simulink library "THAMO_6x2"  (R2018a)
settings: Solver=VariableStepAuto  StartTime=0.0  StopTime=10.0  RelTol=1e-3
undefined symbols (not defined in the file): BM, DiameterLastPiece, DPConstant, DPLinear, DPQuadratic, GeodeticHeight, ID, magnitude, MassFlow, Pressure, Temperature, Water
libraries: carnot x11, simulink x10, $bdroot x3
(part 2 of 3)

== system THAMO_6x2/TVL-Regler mit Hysterese ==
  note: Hystereseregler
      |
      | Erzeuger wird zwischen 0 und 1 mit Hysterese stufig geschalten
  note: Vorlauftemperaturregler
      |
      | Sollvorlauftemperatur wird aus Außentemperatur berechnet, lineares Verhalten zwischen TVLmax bei -16°C und TVLmin bei 20°C (bzw. auch über beide Grenzen hinaus)
  note: Regler Mindestmassenstrom
      |
      | Stellsignal wird nur weitergegeben wenn Massenstrom über Mindestmassenstrom liegt
  note: Reglereinheit Mindestlaufzeit
      |
      | Funktion
      | Maximalwert von Reglerausgang PID und Mindestlaufzeitregler wird gewählt
      | Wert wird geprüft und einem Betriebszustand zugeordnet (1-AN / 0-AUS)
      | IST-Betriebszustand wird integriert - Integrator wird zurückgesetzt, wenn Mindestlaufzeit erreicht
      | Abfrage Wert Integrator, wenn Integrator = 0, wird Stellsignal PID weitergegeben, das =0 sein kann, wenn Mindestlaufzeit nicht erreicht wird Minimalstellsignal ausgegeben
      |
      | Nachteil
      | - Integrator stellt sich immer nach tmin zurück, was dazu führt, dass der Regler immer mindestens tmin als Nachlaufzeit ausgibt
  t_a : Inport
  THB_VL : Inport  Port=2
  Bus Selector : BusSelector  OutputSignals=MassFlow,Temperature
  Compare To Constant : simulink/Logic and Bit Operations/Compare To Constant  relop=>=  const=mmin  OutDataTypeStr=boolean
  Constant : Constant  Value=TVLmax
  Constant1 : Constant  Value=TVLmin
  Constant2 : Constant
  Constant3 : Constant  Value=0
  Constant4 : Constant
  Constant5 : Constant  Value=0
  Constant6 : Constant  Value=T_HG
  Constant7 : Constant
  Integrator : Integrator  ExternalReset=level hold
  Memory : Memory  InitialCondition=1
  MinMax : MinMax  Function=max  Inputs=2
  MinMax1 : MinMax  Function=max  Inputs=2
  Product : Product
  Relay : Relay  OnSwitchValue=hyst_min/2  OffSwitchValue=-hyst_min/2
  Sum : Sum  Inputs=-+|
  Switch1 : Switch  Criteria=u2 > Threshold
  Switch2 : Switch  Threshold=tmin*60
  Switch3 : Switch  Threshold=tmin*60
  Switch4 : Switch  Criteria=u2 > Threshold
  TVL-Regler nach t_a : MATLAB Function  TreatAsAtomicUnit=on
  St : Outport
  wires:
  Memory/1 -> Integrator/2
  Sum/1 -> Relay/1
  TVL-Regler nach t_a/1(TVL_SOLL) -> Sum/2
  Relay/1 -> Product/2  "Stufig"
  Compare To Constant/1 -> Product/1
  Bus Selector/1 -> Compare To Constant/1  "<MassFlow>"
  Product/1 -> MinMax1/1, Switch3/1, Switch4/3, MinMax/1
  Constant1/1 -> TVL-Regler nach t_a/3(TVLmin)
  Constant/1 -> TVL-Regler nach t_a/2(TVLmax)
  t_a/1 -> TVL-Regler nach t_a/1(t_a)
  Bus Selector/2 -> Sum/1  "<Temperature>"
  THB_VL/1 -> Bus Selector/1
  Constant2/1 -> Switch1/1
  Constant3/1 -> Switch1/3
  Switch1/1 -> Integrator/1
  Switch2/1 -> Memory/1
  Constant4/1 -> Switch2/1
  Constant5/1 -> Switch2/3
  Integrator/1 -> Switch2/2, Switch4/2, Switch3/2
  Switch3/1 -> St/1, MinMax/2
  Switch4/1 -> Switch3/3
  MinMax/1 -> Switch1/2
  MinMax1/1 -> Switch4/1
  Constant7/1 -> MinMax1/2
  Constant6/1 -> TVL-Regler nach t_a/4(T_HG)

== system THAMO_6x2/Ventil ==
  note: Ventillaufzeit
  note: Berechnung kv aus St
      | Umrechnung kv in qua
  THB__1_W : Inport
  St : Inport  Port=2
  Bus Assignment : BusAssignment  AssignedSignals=Pressure,DPConstant,DPLinear,DPQuadratic
  Bus Selector : BusSelector  OutputSignals=MassFlow,Pressure
  Bus Selector1 : BusSelector  OutputSignals=DPConstant,DPLinear,DPQuadratic  OutputAsBus=on
  Demux : Demux  Outputs=3
  Rate Limiter : RateLimiter  RisingSlewLimit=1/dt_V  FallingSlewLimit=-1/dt_V  SampleTimeMode=inherited
  Ventilkennlinie : Subsystem
  pressuredrop : Subsystem  mask(pressure drop){}
      mask help:
      | Pressure drop according to input values of con, lin and qua:
      | dp = con + lin*mdot + qua*mdot²
      | The coefficients are also added to the correponding THB elements.
      mask Help: web(fullfile(path_carnot('help'),'Pressuredrop.html'),'-helpbrowser')
  THB__2_W : Outport
  wires:
  Demux/3 -> Bus Assignment/5
  Demux/2 -> Bus Assignment/4
  Bus Selector1/1 -> pressuredrop/3(clq_in)  "clq"
  pressuredrop/1(p_out) -> Bus Assignment/2  "p"
  Bus Selector/1 -> pressuredrop/1(mdot)  "<MassFlow>"
  Bus Selector/2 -> pressuredrop/2(p_in)  "<Pressure>"
  pressuredrop/2(clq_out) -> Demux/1  "clq"
  St/1 -> Rate Limiter/1
  THB__1_W/1 -> Bus Selector1/1, Ventilkennlinie/2(THB__1_W), Bus Selector/1, Bus Assignment/1
  Bus Assignment/1 -> THB__2_W/1
  Demux/1 -> Bus Assignment/3
  Ventilkennlinie/1(qua) -> pressuredrop/4(qua)
  Rate Limiter/1 -> Ventilkennlinie/1(St)

== system THAMO_6x2/Verbraucher_RK-Modell ==
  T___L : Inport
  THB__1_W : Inport  Port=2
  HK_MST_Ruehrkesselkask : Subsystem  mask(Heizkoerper als Ruehrkesselkaskade){}
      mask help:
      | Modell aus MST der HBC
      | Rührkesselkaskade aus 3 Elementen
  Pressure_Drop : Subsystem  mask(fixed pressure drop){}
      mask help:
      | Constant parameters for pressure drop in a flow.
      | dp = c + l*mdot + q*mdot²
      | Calculation is done for ID > 10000 (dp = f(l, q), c is neglected) and ID > 20000 (dp = f(c,l,q)).
      | Applied directly to the THB bus.
      mask Help: web(fullfile(path_carnot('help'),'Pressure_Drop_Fix.html'),'-helpbrowser')
  Qdot : Outport
  THB__2_W : Outport  Port=2
  wires:
  HK_MST_Ruehrkesselkask/2(Qdot_2) -> Qdot/1
  T___L/1 -> HK_MST_Ruehrkesselkask/2(t__L)
  THB__1_W/1 -> HK_MST_Ruehrkesselkask/1(THB__1_W)
  HK_MST_Ruehrkesselkask/1(THB__2_W) -> Pressure_Drop/1(THB__1_W)
  Pressure_Drop/1(THB__2_W) -> THB__2_W/1

== system THAMO_6x2/Wärmeabnehmer ==
  note: Wärmeabgabe
      |
      |
      |
      |
      |
      |
      |
      |
      |
      |
      | T_RL aus Leistung lädt/entlädt Kapazität des WA
  THB__1_W : Inport
  Qdot_2 in W : Inport  Port=2
  Pressure_Drop : Subsystem  mask(fixed pressure drop){}
      mask help:
      | Constant parameters for pressure drop in a flow.
      | dp = c + l*mdot + q*mdot²
      | Calculation is done for ID > 10000 (dp = f(l, q), c is neglected) and ID > 20000 (dp = f(c,l,q)).
      | Applied directly to the THB bus.
      mask Help: web(fullfile(path_carnot('help'),'Pressure_Drop_Fix.html'),'-helpbrowser')
  Temperatur : Subsystem
  THB__2_W : Outport
  wires:
  Pressure_Drop/1(THB__2_W) -> THB__2_W/1
  Temperatur/1(THB__2_W) -> Pressure_Drop/1(THB__1_W)
  Qdot_2 in W/1 -> Temperatur/2(Qdot_2)
  THB__1_W/1 -> Temperatur/1(THB__1_W)

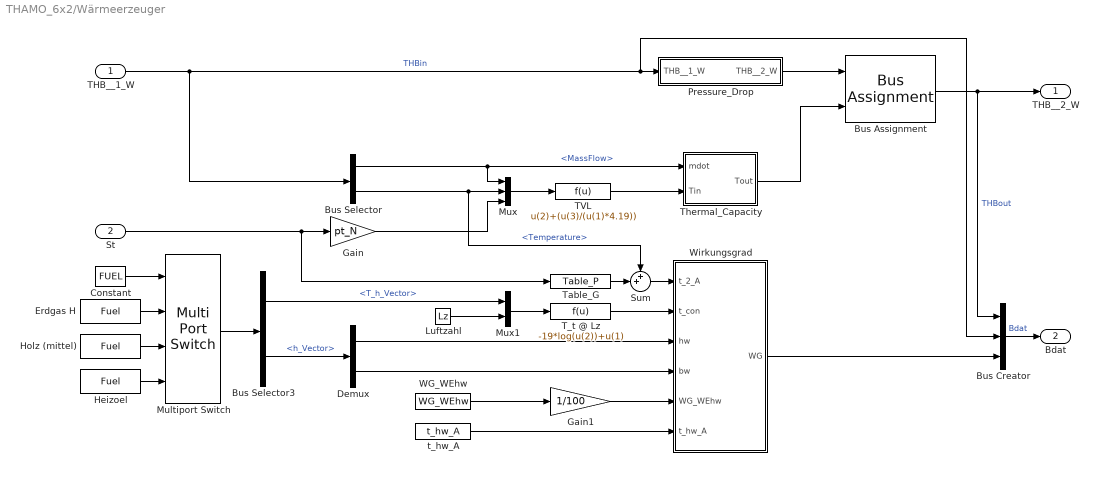
== system THAMO_6x2/Wärmeerzeuger ==
  THB__1_W : Inport
  St : Inport  Port=2
  Bus Assignment : BusAssignment  AssignedSignals=Temperature
  Bus Creator : BusCreator  Inputs=3
  Bus Selector : BusSelector  OutputSignals=MassFlow,Temperature
  Bus Selector3 : BusSelector  OutputSignals=T_h_Vector,h_Vector
  Constant : Constant  Value=FUEL
  Demux : Demux  Outputs=2
  Erdgas H : carnot/Source/Energy/Fuel  ft=1  t=20  ls=15.59  p=1e5  h_values=[38.5 43]*10^6  tc=57.53  price=1  mass=[0.22 0.70 0.05 0 0.03 0]
  Gain : Gain  Gain=pt_N
  Gain1 : Gain  Gain=1/100
  Heizoel : carnot/Source/Energy/Fuel  ft=2  t=20  ls=15.94  p=1e5  h_values=[42.6 45.4]*10^6  tc=50.37  price=1  mass=[0.13 0.87 0 0 0 0]
  Holz (mittel) : carnot/Source/Energy/Fuel  ft=3  t=20  ls=6.54  p=1e5  h_values=[15.1 19]*10^6  tc=67.5  price=1  mass=[0.06 0.5 0.44 0 0 0]
  Luftzahl : Constant  Value=Lz
  Multiport Switch : MultiPortSwitch
  Mux : Mux  Inputs=3
  Mux1 : Mux  Inputs=2
  Pressure_Drop : Subsystem  mask(fixed pressure drop){}
      mask help:
      | Constant parameters for pressure drop in a flow.
      | dp = c + l*mdot + q*mdot²
      | Calculation is done for ID > 10000 (dp = f(l, q), c is neglected) and ID > 20000 (dp = f(c,l,q)).
      | Applied directly to the THB bus.
      mask Help: web(fullfile(path_carnot('help'),'Pressure_Drop_Fix.html'),'-helpbrowser')
  Sum : Sum  Inputs=++|
  TVL : Fcn  Expr=u(2)+(u(3)/(u(1)*4.19))
  T_t @ Lz : Fcn  Expr=-19*log(u(2))+u(1)
  Table_G : $bdroot/Brennwertkessel/Table_P  NumberOfTableDimensions=1  DataSpecification=Table and breakpoints  BreakpointsSpecification=Explicit values  BreakpointsForDimension1=[0 0.5 1]  BreakpointsForDimension2=[10,22,31]  BreakpointsForDimension3=[1:3]  BreakpointsForDimension4=[1:3]  BreakpointsForDimension5=[1:3]  BreakpointsForDimension6=[1:3]  BreakpointsForDimension7=[1:3]  BreakpointsForDimension8=[1:3]  BreakpointsForDimension9=[1:3]  BreakpointsForDimension10=[1:3]  BreakpointsForDimension11=[1:3]  BreakpointsForDimension12=[1:3]  BreakpointsForDimension13=[1:3]  BreakpointsForDimension14=[1:3]  BreakpointsForDimension15=[1:3]  BreakpointsForDimension16=[1:3]  BreakpointsForDimension17=[1:3]  BreakpointsForDimension18=[1:3]  BreakpointsForDimension19=[1:3]  BreakpointsForDimension20=[1:3]  BreakpointsForDimension21=[1:3]  BreakpointsForDimension22=[1:3]  BreakpointsForDimension23=[1:3]  BreakpointsForDimension24=[1:3]  BreakpointsForDimension25=[1:3]  BreakpointsForDimension26=[1:3]  BreakpointsForDimension27=[1:3]  BreakpointsForDimension28=[1:3]  BreakpointsForDimension29=[1:3]  BreakpointsForDimension30=[1:3]  BreakpointsForDimension1FirstPoint=1  BreakpointsForDimension2FirstPoint=1  BreakpointsForDimension3FirstPoint=1  BreakpointsForDimension4FirstPoint=1  BreakpointsForDimension5FirstPoint=1  BreakpointsForDimension6FirstPoint=1  BreakpointsForDimension7FirstPoint=1  BreakpointsForDimension8FirstPoint=1  BreakpointsForDimension9FirstPoint=1  BreakpointsForDimension10FirstPoint=1  BreakpointsForDimension11FirstPoint=1  BreakpointsForDimension12FirstPoint=1  BreakpointsForDimension13FirstPoint=1  BreakpointsForDimension14FirstPoint=1  BreakpointsForDimension15FirstPoint=1  BreakpointsForDimension16FirstPoint=1  BreakpointsForDimension17FirstPoint=1  BreakpointsForDimension18FirstPoint=1  BreakpointsForDimension19FirstPoint=1  BreakpointsForDimension20FirstPoint=1  BreakpointsForDimension21FirstPoint=1  BreakpointsForDimension22FirstPoint=1  BreakpointsForDimension23FirstPoint=1  BreakpointsForDimension24FirstPoint=1  BreakpointsForDimension25FirstPoint=1  BreakpointsForDimension26FirstPoint=1  BreakpointsForDimension27FirstPoint=1  BreakpointsForDimension28FirstPoint=1  BreakpointsForDimension29FirstPoint=1  BreakpointsForDimension30FirstPoint=1  BreakpointsForDimension1Spacing=1  BreakpointsForDimension2Spacing=1  BreakpointsForDimension3Spacing=1  BreakpointsForDimension4Spacing=1  BreakpointsForDimension5Spacing=1  BreakpointsForDimension6Spacing=1  BreakpointsForDimension7Spacing=1  BreakpointsForDimension8Spacing=1  BreakpointsForDimension9Spacing=1  BreakpointsForDimension10Spacing=1  BreakpointsForDimension11Spacing=1  BreakpointsForDimension12Spacing=1  BreakpointsForDimension13Spacing=1  BreakpointsForDimension14Spacing=1  BreakpointsForDimension15Spacing=1  BreakpointsForDimension16Spacing=1  BreakpointsForDimension17Spacing=1  BreakpointsForDimension18Spacing=1  BreakpointsForDimension19Spacing=1  BreakpointsForDimension20Spacing=1  BreakpointsForDimension21Spacing=1  BreakpointsForDimension22Spacing=1  BreakpointsForDimension23Spacing=1  BreakpointsForDimension24Spacing=1  BreakpointsForDimension25Spacing=1  BreakpointsForDimension26Spacing=1  BreakpointsForDimension27Spacing=1  BreakpointsForDimension28Spacing=1  BreakpointsForDimension29Spacing=1  BreakpointsForDimension30Spacing=1  BreakpointsForDimension1Min=[]  BreakpointsForDimension2Min=[]  BreakpointsForDimension3Min=[]  BreakpointsForDimension4Min=[]  BreakpointsForDimension5Min=[]  BreakpointsForDimension6Min=[]  BreakpointsForDimension7Min=[]  BreakpointsForDimension8Min=[]  BreakpointsForDimension9Min=[]  BreakpointsForDimension10Min=[]  BreakpointsForDimension11Min=[]  BreakpointsForDimension12Min=[]  BreakpointsForDimension13Min=[]  BreakpointsForDimension14Min=[]  BreakpointsForDimension15Min=[]  BreakpointsForDimension16Min=[]  BreakpointsForDimension17Min=[]  BreakpointsForDimension18Min=[]  BreakpointsForDimension19Min=[]  BreakpointsForDimension20Min=[]  BreakpointsForDimension21Min=[]  BreakpointsForDimension22Min=[]  BreakpointsForDimension23Min=[]  BreakpointsForDimension24Min=[]  BreakpointsForDimension25Min=[]  BreakpointsForDimension26Min=[]  BreakpointsForDimension27Min=[]  BreakpointsForDimension28Min=[]  BreakpointsForDimension29Min=[]  BreakpointsForDimension30Min=[]  BreakpointsForDimension1Max=[]  BreakpointsForDimension2Max=[]  BreakpointsForDimension3Max=[]  BreakpointsForDimension4Max=[]  BreakpointsForDimension5Max=[]  BreakpointsForDimension6Max=[]  BreakpointsForDimension7Max=[]  BreakpointsForDimension8Max=[]  BreakpointsForDimension9Max=[]  BreakpointsForDimension10Max=[]  BreakpointsForDimension11Max=[]  BreakpointsForDimension12Max=[]  BreakpointsForDimension13Max=[]  BreakpointsForDimension14Max=[]  BreakpointsForDimension15Max=[]  BreakpointsForDimension16Max=[]  BreakpointsForDimension17Max=[]  BreakpointsForDimension18Max=[]  BreakpointsForDimension19Max=[]  BreakpointsForDimension20Max=[]  BreakpointsForDimension21Max=[]  BreakpointsForDimension22Max=[]  BreakpointsForDimension23Max=[]  BreakpointsForDimension24Max=[]  BreakpointsForDimension25Max=[]  BreakpointsForDimension26Max=[]  BreakpointsForDimension27Max=[]  BreakpointsForDimension28Max=[]  BreakpointsForDimension29Max=[]  BreakpointsForDimension30Max=[]  BreakpointsForDimension1DataTypeStr=Inherit: Same as corresponding input  BreakpointsForDimension2DataTypeStr=Inherit: Same as corresponding input  BreakpointsForDimension3DataTypeStr=Inherit: Same as corresponding input  BreakpointsForDimension4DataTypeStr=Inherit: Same as corresponding input  BreakpointsForDimension5DataTypeStr=Inherit: Same as corresponding input  BreakpointsForDimension6DataTypeStr=Inherit: Same as corresponding input  BreakpointsForDimension7DataTypeStr=Inherit: Same as corresponding input  BreakpointsForDimension8DataTypeStr=Inherit: Same as corresponding input  BreakpointsForDimension9DataTypeStr=Inherit: Same as corresponding input  BreakpointsForDimension10DataTypeStr=Inherit: Same as corresponding input  BreakpointsForDimension11DataTypeStr=Inherit: Same as corresponding input  BreakpointsForDimension12DataTypeStr=Inherit: Same as corresponding input  BreakpointsForDimension13DataTypeStr=Inherit: Same as corresponding input  BreakpointsForDimension14DataTypeStr=Inherit: Same as corresponding input  BreakpointsForDimension15DataTypeStr=Inherit: Same as corresponding input  BreakpointsForDimension16DataTypeStr=Inherit: Same as corresponding input  BreakpointsForDimension17DataTypeStr=Inherit: Same as corresponding input  BreakpointsForDimension18DataTypeStr=Inherit: Same as corresponding input  BreakpointsForDimension19DataTypeStr=Inherit: Same as corresponding input  BreakpointsForDimension20DataTypeStr=Inherit: Same as corresponding input  BreakpointsForDimension21DataTypeStr=Inherit: Same as corresponding input  BreakpointsForDimension22DataTypeStr=Inherit: Same as corresponding input  BreakpointsForDimension23DataTypeStr=Inherit: Same as corresponding input  BreakpointsForDimension24DataTypeStr=Inherit: Same as corresponding input  BreakpointsForDimension25DataTypeStr=Inherit: Same as corresponding input  BreakpointsForDimension26DataTypeStr=Inherit: Same as corresponding input  BreakpointsForDimension27DataTypeStr=Inherit: Same as corresponding input  BreakpointsForDimension28DataTypeStr=Inherit: Same as corresponding input  BreakpointsForDimension29DataTypeStr=Inherit: Same as corresponding input  BreakpointsForDimension30DataTypeStr=Inherit: Same as corresponding input  IndexSearchMethod=Binary search  BeginIndexSearchUsingPreviousIndexResult=off  UseOneInputPortForAllInputData=off  Table=[0 G]  TableMin=[]  TableMax=[]  TableDataTypeStr=Inherit: Same as output  IntermediateResultsDataTypeStr=Inherit: Same as output  InterpMethod=Linear point-slope  ExtrapMethod=Linear  DiagnosticForOutOfRangeInput=None  RemoveProtectionInput=off  UseLastTableValue=off  SampleTime=-1  InternalRulePriority=Speed  InputSameDT=on  OutMin=[]  OutMax=[]  SupportTunableTableSize=off  MaximumIndicesForEachDimension=[]
  Thermal_Capacity : Subsystem  mask(Thermal Capacity){}
      mask help: Basic one node model of a thermal mass using the differential equation:
      mask Help: web(fullfile(path_carnot('help'),'Thermal_Capacity.html'),'-helpbrowser')
  WG_WEhw : Constant  Value=WG_WEhw
  Wirkungsgrad : MATLAB Function  TreatAsAtomicUnit=on
  t_hw_A : Constant  Value=t_hw_A
  THB__2_W : Outport
  Bdat : Outport  Port=2
  wires:
  Pressure_Drop/1(THB__2_W) -> Bus Assignment/1
  Bus Assignment/1 -> Bus Creator/1, THB__2_W/1  "THBout"
  THB__1_W/1 -> Bus Creator/2, Pressure_Drop/1(THB__1_W), Bus Selector/1  "THBin"
  Thermal_Capacity/1(Tout) -> Bus Assignment/2
  Bus Selector/1 -> Thermal_Capacity/1(mdot), Mux/1  "<MassFlow>"
  St/1 -> Table_G/1, Gain/1
  Gain/1 -> Mux/3
  Bus Selector/2 -> Sum/1, Mux/2  "<Temperature>"
  Mux/1 -> TVL/1
  TVL/1 -> Thermal_Capacity/2(Tin)
  t_hw_A/1 -> Wirkungsgrad/6(t_hw_A)
  T_t @ Lz/1 -> Wirkungsgrad/2(t_con)
  Bus Selector3/2 -> Demux/1  "<h_Vector>"
  Demux/1 -> Wirkungsgrad/3(hw)
  Demux/2 -> Wirkungsgrad/4(bw)
  Mux1/1 -> T_t @ Lz/1
  WG_WEhw/1 -> Gain1/1
  Gain1/1 -> Wirkungsgrad/5(WG_WEhw)
  Bus Selector3/1 -> Mux1/1  "<T_h_Vector>"
  Luftzahl/1 -> Mux1/2
  Heizoel/1 -> Multiport Switch/4
  Erdgas H/1 -> Multiport Switch/2
  Holz (mittel)/1 -> Multiport Switch/3
  Constant/1 -> Multiport Switch/1
  Multiport Switch/1 -> Bus Selector3/1
  Sum/1 -> Wirkungsgrad/1(t_2_A)
  Table_G/1 -> Sum/2
  Bus Creator/1 -> Bdat/1  "Bdat"
  Wirkungsgrad/1(WG) -> Bus Creator/3

== system THAMO_6x2/Überströmventil ==
  THB__1_W : Inport
  Bus Assignment : BusAssignment  AssignedSignals=Pressure,DPConstant,DPLinear,DPQuadratic
  Bus Selector : BusSelector  OutputSignals=MassFlow,Pressure
  Bus Selector1 : BusSelector  OutputSignals=DPConstant,DPLinear,DPQuadratic  OutputAsBus=on
  Constant1 : Constant  Value=p0
  Constant2 : Constant  Value=p1
  Constant3 : Constant  Value=p2
  Demux : Demux  Outputs=3
  pressuredrop : Subsystem  mask(pressure drop){}
      mask help:
      | Pressure drop according to input values of con, lin and qua:
      | dp = con + lin*mdot + qua*mdot²
      | The coefficients are also added to the correponding THB elements.
      mask Help: web(fullfile(path_carnot('help'),'Pressuredrop.html'),'-helpbrowser')
  THB__2_W : Outport
  wires:
  Demux/3 -> Bus Assignment/5
  Demux/2 -> Bus Assignment/4
  Demux/1 -> Bus Assignment/3
  Bus Assignment/1 -> THB__2_W/1
  THB__1_W/1 -> Bus Selector1/1, Bus Selector/1, Bus Assignment/1
  pressuredrop/2(clq_out) -> Demux/1  "clq"
  Bus Selector/2 -> pressuredrop/2(p_in)  "<Pressure>"
  Bus Selector/1 -> pressuredrop/1(mdot)  "<MassFlow>"
  pressuredrop/1(p_out) -> Bus Assignment/2  "p"
  Bus Selector1/1 -> pressuredrop/3(clq_in)  "clq"
  Constant1/1 -> pressuredrop/4(con)
  Constant2/1 -> pressuredrop/5(lin)
  Constant3/1 -> pressuredrop/6(qua)

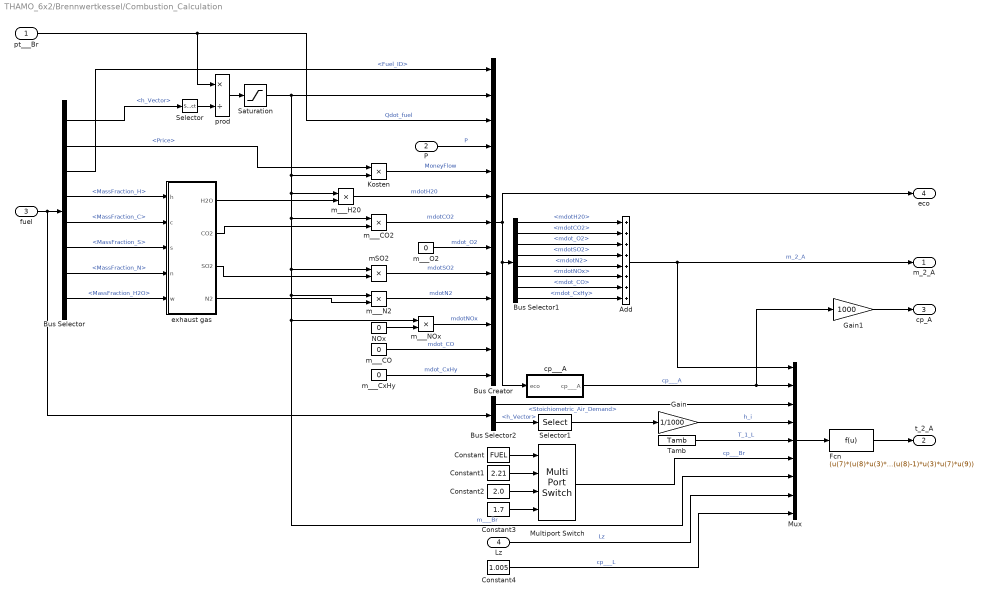
== system THAMO_6x2/Brennwertkessel/Combustion_Calculation ==
  pt___Br : Inport
  P : Inport  Port=2
  fuel : Inport  Port=3
  Lz : Inport  Port=4
  Add : Sum  Inputs=++++++++
  Bus Creator : BusCreator  Inputs=13
  Bus Selector : BusSelector  OutputSignals=h_Vector,Price,Fuel_ID,MassFraction_H,MassFraction_C,MassFraction_S,MassFraction_N,MassFraction_H2O
  Bus Selector1 : BusSelector  OutputSignals=mdotH20,mdotCO2,mdot_O2,mdotSO2,mdotN2,mdotNOx,mdot_CO,mdot_CxHy
  Bus Selector2 : BusSelector  OutputSignals=Stoichiometric_Air_Demand,h_Vector
  Constant : Constant  Value=FUEL
  Constant1 : Constant  Value=2.21
  Constant2 : Constant  Value=2.0
  Constant3 : Constant  Value=1.7
  Constant4 : Constant  Value=1.005
  Fcn : Fcn  Expr=(u(7)*(u(8)*u(3)*u(9)*u(5)+u(6)*u(5)+u(4)))/(u(1)*u(2)+(u(8)-1)*u(3)*u(7)*u(9))
  Gain : Gain  Gain=1/1000
  Gain1 : Gain  Gain=1000
  Kosten : Product  SaturateOnIntegerOverflow=on  InputSameDT=on  OutDataTypeStr=Inherit: Same as first input
  Multiport Switch : MultiPortSwitch
  Mux : Mux  Inputs=9
  NOx : Constant  Value=0
  Saturation : Saturate  UpperLimit=inf  LowerLimit=10^-20
  Selector : Selector  IndexOptions=Index vector (dialog)  Indices=[1]  OutputSizes=1
  Selector1 : Selector  IndexOptions=Index vector (dialog)  Indices=[1]  OutputSizes=1
  Tamb : Constant  Value=Tamb
  cp___A : Subsystem
  exhaust gas : Subsystem
  mSO2 : Product  SaturateOnIntegerOverflow=on  InputSameDT=on  OutDataTypeStr=Inherit: Same as first input
  m___CO : Constant  Value=0
  m___CO2 : Product  SaturateOnIntegerOverflow=on  InputSameDT=on  OutDataTypeStr=Inherit: Same as first input
  m___CxHy : Constant  Value=0
  m___H20 : Product  SaturateOnIntegerOverflow=on  InputSameDT=on  OutDataTypeStr=Inherit: Same as first input
  m___N2 : Product  SaturateOnIntegerOverflow=on  InputSameDT=on  OutDataTypeStr=Inherit: Same as first input
  m___NOx : Product  SaturateOnIntegerOverflow=on  InputSameDT=on  OutDataTypeStr=Inherit: Same as first input
  m___O2 : Constant  Value=0
  prod : Product  Inputs=*/  SaturateOnIntegerOverflow=on  InputSameDT=on  OutDataTypeStr=Inherit: Same as first input
  m_2_A : Outport  InitialOutput=0
  t_2_A : Outport  Port=2  InitialOutput=0
  cp_A : Outport  Port=3  InitialOutput=0
  eco : Outport  Port=4  InitialOutput=0
  wires:
  Saturation/1 -> m___N2/1, m___NOx/1, Mux/7, mSO2/1, m___CO2/1, m___H20/1, Kosten/2, Bus Creator/2  "m___Br"
  cp___A/1(cp___A) -> Gain1/1, Mux/2  "cp___A"
  Constant4/1 -> Mux/9  "cp___L"
  Tamb/1 -> Mux/5  "T_1_L"
  Gain/1 -> Mux/4  "h_i"
  Mux/1 -> Fcn/1
  Selector1/1 -> Gain/1
  Lz/1 -> Mux/8  "Lz"
  Multiport Switch/1 -> Mux/6  "cp___Br"
  Constant3/1 -> Multiport Switch/4
  Constant2/1 -> Multiport Switch/3
  Constant1/1 -> Multiport Switch/2
  Constant/1 -> Multiport Switch/1
  Bus Selector2/1 -> Mux/3  "<Stoichiometric_Air_Demand>"
  Bus Selector2/2 -> Selector1/1  "<h_Vector>"
  Add/1 -> m_2_A/1, Mux/1  "m_2_A"
  Bus Selector1/8 -> Add/8  "<mdot_CxHy>"
  Bus Selector1/7 -> Add/7  "<mdot_CO>"
  Bus Selector1/6 -> Add/6  "<mdotNOx>"
  Bus Selector1/5 -> Add/5  "<mdotN2>"
  Bus Selector1/4 -> Add/4  "<mdotSO2>"
  Bus Selector1/3 -> Add/3  "<mdot_O2>"
  Bus Selector1/2 -> Add/2  "<mdotCO2>"
  Bus Selector1/1 -> Add/1  "<mdotH20>"
  pt___Br/1 -> Bus Creator/3, prod/1  "Qdot_fuel"
  m___N2/1 -> Bus Creator/10  "mdotN2"
  exhaust gas/1(H2O) -> m___H20/2
  exhaust gas/2(CO2) -> m___CO2/2
  exhaust gas/4(N2) -> m___N2/2
  NOx/1 -> m___NOx/2
  exhaust gas/3(SO2) -> mSO2/2
  Bus Selector/8 -> exhaust gas/5(w)  "<MassFraction_H2O>"
  Bus Selector/7 -> exhaust gas/4(n)  "<MassFraction_N>"
  Bus Selector/6 -> exhaust gas/3(s)  "<MassFraction_S>"
  Bus Selector/5 -> exhaust gas/2(c)  "<MassFraction_C>"
  Bus Selector/4 -> exhaust gas/1(h)  "<MassFraction_H>"
  Bus Selector/3 -> Bus Creator/1  "<Fuel_ID>"
  prod/1 -> Saturation/1
  Bus Selector/2 -> Kosten/1  "<Price>"
  m___CxHy/1 -> Bus Creator/13  "mdot_CxHy"
  m___CO/1 -> Bus Creator/12  "mdot_CO"
  m___NOx/1 -> Bus Creator/11  "mdotNOx"
  mSO2/1 -> Bus Creator/9  "mdotSO2"
  m___O2/1 -> Bus Creator/8  "mdot_O2"
  m___CO2/1 -> Bus Creator/7  "mdotCO2"
  m___H20/1 -> Bus Creator/6  "mdotH20"
  Kosten/1 -> Bus Creator/5  "MoneyFlow"
  P/1 -> Bus Creator/4  "P"
  Bus Selector/1 -> Selector/1  "<h_Vector>"
  fuel/1 -> Bus Selector/1, Bus Selector2/1
  Selector/1 -> prod/2
  Bus Creator/1 -> eco/1, Bus Selector1/1, cp___A/1(eco)
  Gain1/1 -> cp_A/1
  Fcn/1 -> t_2_A/1

== system THAMO_6x2/Brennwertkessel/Pressure_Drop ==
  THB__1_W : Inport
  Bus Assignment1 : BusAssignment  AssignedSignals=Pressure,DPConstant,DPLinear,DPQuadratic
  Bus Selector3 : BusSelector  OutputSignals=MassFlow,Pressure
  Bus Selector4 : BusSelector  OutputSignals=DPConstant,DPLinear,DPQuadratic  OutputAsBus=on
  Bus Selector5 : BusSelector  OutputSignals=ID
  Compare To Constant1 : simulink/Logic and Bit Operations/Compare To Constant  relop=>  const=0  OutDataTypeStr=boolean
  Demux2 : Demux  Outputs=3
  Pressuredrop : carnot/Basic/Pressure_Drop/Pressuredrop
  lq_calc : Subsystem
  THB__2_W : Outport
  wires:
  Compare To Constant1/1 -> lq_calc/Enable
  lq_calc/1(qua) -> Pressuredrop/4
  Demux2/3 -> Bus Assignment1/5
  Demux2/2 -> Bus Assignment1/4
  Demux2/1 -> Bus Assignment1/3
  Bus Assignment1/1 -> THB__2_W/1
  Pressuredrop/1 -> Bus Assignment1/2
  THB__1_W/1 -> Bus Selector5/1, lq_calc/1(THB__1_W), Bus Selector4/1, Bus Selector3/1, Bus Assignment1/1
  Bus Selector4/1 -> Pressuredrop/3
  Bus Selector3/1 -> Pressuredrop/1  "<MassFlow>"
  Bus Selector3/2 -> Pressuredrop/2  "<Pressure>"
  Bus Selector5/1 -> Compare To Constant1/1  "<ID>"
  Pressuredrop/2 -> Demux2/1

== system THAMO_6x2/Brennwertkessel/Subsystem ==
  WG : Inport
  eco_in : Inport  Port=2
  Bus Creator : BusCreator  Inputs=14
  Bus Selector : BusSelector  OutputSignals=Fuel_ID,m___Br,Qdot_fuel,P,MoneyFlow,mdotH20,mdotCO2,mdot_O2,mdotSO2,mdotN2,mdotNOx,mdot_CO,mdot_CxHy
  eco : Outport
  wires:
  eco_in/1 -> Bus Selector/1
  Bus Creator/1 -> eco/1  "eco"
  Bus Selector/2 -> Bus Creator/2  "<m___Br>"
  Bus Selector/1 -> Bus Creator/1  "<Fuel_ID>"
  Bus Selector/3 -> Bus Creator/3  "<Qdot_fuel>"
  Bus Selector/4 -> Bus Creator/4  "<P>"
  Bus Selector/5 -> Bus Creator/5  "<MoneyFlow>"
  Bus Selector/6 -> Bus Creator/6  "<mdotH20>"
  Bus Selector/7 -> Bus Creator/7  "<mdotCO2>"
  Bus Selector/8 -> Bus Creator/8  "<mdot_O2>"
  Bus Selector/9 -> Bus Creator/9  "<mdotSO2>"
  Bus Selector/10 -> Bus Creator/10  "<mdotN2>"
  Bus Selector/11 -> Bus Creator/11  "<mdotNOx>"
  Bus Selector/12 -> Bus Creator/12  "<mdot_CO>"
  Bus Selector/13 -> Bus Creator/13  "<mdot_CxHy>"
  WG/1 -> Bus Creator/14

== system THAMO_6x2/Brennwertkessel/Thermal_Capacity ==
  mdot : Inport
  Tin : Inport  Port=2
  Divide : Product  Inputs=*/
  Integrator : Integrator  InitialCondition=Tamb
  Losses : Gain  Gain=UV  SaturateOnIntegerOverflow=on  OutDataTypeStr=Inherit: Same as input  ParamDataTypeStr=Inherit: Same as input
  Product1 : Product  Inputs=3  SaturateOnIntegerOverflow=on  InputSameDT=on  OutDataTypeStr=Inherit: Same as first input
  Product3 : Product  Inputs=3  SaturateOnIntegerOverflow=on  InputSameDT=on  OutDataTypeStr=Inherit: Same as first input
  Sum1 : Sum  Inputs=-+  SaturateOnIntegerOverflow=on  InputSameDT=on  OutDataTypeStr=Inherit: Same as first input
  Sum2 : Sum  Inputs=-+  SaturateOnIntegerOverflow=on  InputSameDT=on  OutDataTypeStr=Inherit: Same as first input
  Sum3 : Sum  Inputs=+-  SaturateOnIntegerOverflow=on  InputSameDT=on  OutDataTypeStr=Inherit: Same as first input
  Tamb : Constant  Value=Tamb
  Tamb1 : Constant  Value=V/2
  cp : Lookup_n-D  NumberOfTableDimensions=1  BreakpointsForDimension1=[0,10,20,30,40,50,60,70,80,90,100]  Table=[4218,4192,4182,4179,4179,4181,4184,4190,4196,4205,4216]  InternalRulePriority=Speed  RndMeth=Simplest  InputSameDT=on
  rho : Lookup_n-D  NumberOfTableDimensions=1  BreakpointsForDimension1=[0,10,20,30,40,50,60,70,80,90,100]  Table=[999.84,999.7,998.2,995.64,992.21,988.03,983.19,977.76,971.79,965.3,958.35]  InternalRulePriority=Speed  RndMeth=Simplest  InputSameDT=on
  Tout : Outport
  wires:
  Tamb1/1 -> Product3/3
  rho/1 -> Product3/2
  Product3/1 -> Divide/2
  Tin/1 -> Sum1/2
  Sum1/1 -> Product1/1
  Divide/1 -> Integrator/1
  cp/1 -> Product1/3, Product3/1
  Sum3/1 -> Losses/1
  Losses/1 -> Sum2/1
  Tamb/1 -> Sum3/2
  Sum2/1 -> Divide/1
  Product1/1 -> Sum2/2
  Integrator/1 -> Tout/1, Sum3/1, Sum1/1, cp/1, rho/1
  mdot/1 -> Product1/2

== system THAMO_6x2/Brennwertkessel/Thermal_Capacity1 ==
  mdot : Inport
  Tin : Inport  Port=2
  Divide : Product  Inputs=*/
  Integrator : Integrator  InitialCondition=Tamb
  Losses : Gain  Gain=UV  SaturateOnIntegerOverflow=on  OutDataTypeStr=Inherit: Same as input  ParamDataTypeStr=Inherit: Same as input
  Product1 : Product  Inputs=3  SaturateOnIntegerOverflow=on  InputSameDT=on  OutDataTypeStr=Inherit: Same as first input
  Product3 : Product  Inputs=3  SaturateOnIntegerOverflow=on  InputSameDT=on  OutDataTypeStr=Inherit: Same as first input
  Sum1 : Sum  Inputs=-+  SaturateOnIntegerOverflow=on  InputSameDT=on  OutDataTypeStr=Inherit: Same as first input
  Sum2 : Sum  Inputs=-+  SaturateOnIntegerOverflow=on  InputSameDT=on  OutDataTypeStr=Inherit: Same as first input
  Sum3 : Sum  Inputs=+-  SaturateOnIntegerOverflow=on  InputSameDT=on  OutDataTypeStr=Inherit: Same as first input
  Tamb : Constant  Value=Tamb
  Tamb1 : Constant  Value=V/2
  cp : Lookup_n-D  NumberOfTableDimensions=1  BreakpointsForDimension1=[0,10,20,30,40,50,60,70,80,90,100]  Table=[4218,4192,4182,4179,4179,4181,4184,4190,4196,4205,4216]  InternalRulePriority=Speed  RndMeth=Simplest  InputSameDT=on
  rho : Lookup_n-D  NumberOfTableDimensions=1  BreakpointsForDimension1=[0,10,20,30,40,50,60,70,80,90,100]  Table=[999.84,999.7,998.2,995.64,992.21,988.03,983.19,977.76,971.79,965.3,958.35]  InternalRulePriority=Speed  RndMeth=Simplest  InputSameDT=on
  Tout : Outport
  wires:
  Tamb1/1 -> Product3/3
  rho/1 -> Product3/2
  Product3/1 -> Divide/2
  Tin/1 -> Sum1/2
  Sum1/1 -> Product1/1
  Divide/1 -> Integrator/1
  cp/1 -> Product1/3, Product3/1
  Sum3/1 -> Losses/1
  Losses/1 -> Sum2/1
  Tamb/1 -> Sum3/2
  Sum2/1 -> Divide/1
  Product1/1 -> Sum2/2
  Integrator/1 -> rho/1, cp/1, Tout/1, Sum3/1, Sum1/1
  mdot/1 -> Product1/2

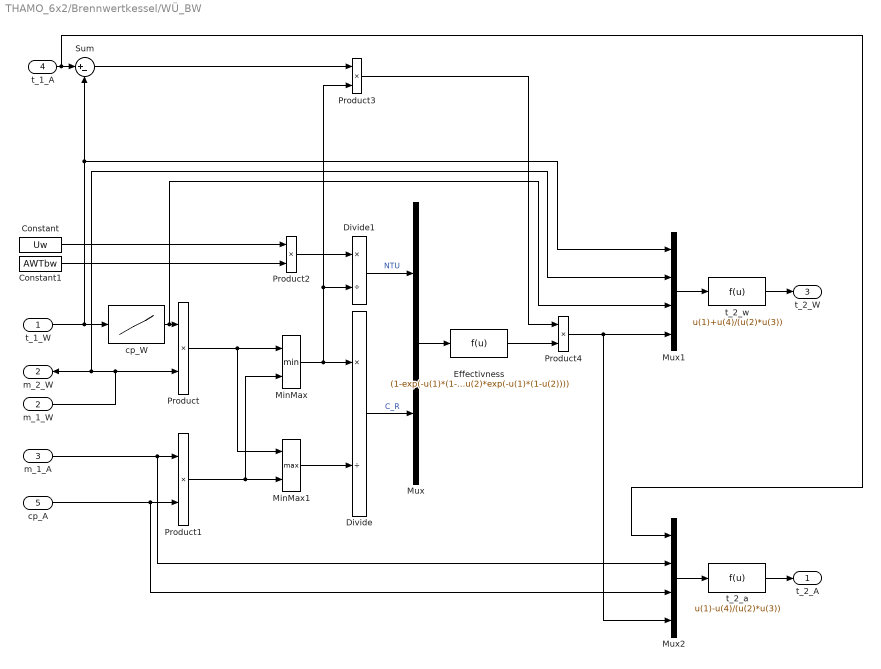
== system THAMO_6x2/Brennwertkessel/WÜ_BW ==
  t_1_W : Inport
  m_1_W : Inport  Port=2
  m_1_A : Inport  Port=3
  t_1_A : Inport  Port=4
  cp_A : Inport  Port=5
  Constant : Constant  Value=Uw
  Constant1 : Constant  Value=AWTbw
  Divide : Product  Inputs=*/
  Divide1 : Product  Inputs=*/
  Effectivness : Fcn  Expr=(1-exp(-u(1)*(1-u(2))))/(1-u(2)*exp(-u(1)*(1-u(2))))
  MinMax : MinMax  Inputs=2
  MinMax1 : MinMax  Function=max  Inputs=2
  Mux : Mux  Inputs=2
  Mux1 : Mux
  Mux2 : Mux
  Product{,1..4} (5 alike) : Product
  Sum : Sum  Inputs=|+-
  cp_W : Lookup_n-D  NumberOfTableDimensions=1  BreakpointsForDimension1=[0,10,20,30,40,50,60,70,80,90,100]  Table=[4218,4192,4182,4179,4179,4181,4184,4190,4196,4205,4216]  InternalRulePriority=Speed  RndMeth=Simplest  InputSameDT=on
  t_2_a : Fcn  Expr=u(1)-u(4)/(u(2)*u(3))
  t_2_w : Fcn  Expr=u(1)+u(4)/(u(2)*u(3))
  t_2_A : Outport
  m_2_W : Outport  Port=2
  t_2_W : Outport  Port=3
  wires:
  t_1_W/1 -> cp_W/1, Mux1/1, Sum/2
  cp_W/1 -> Mux1/3, Product/1
  m_1_A/1 -> Mux2/2, Product1/1
  cp_A/1 -> Mux2/3, Product1/2
  Product/1 -> MinMax1/1, MinMax/1
  Product1/1 -> MinMax/2, MinMax1/2
  MinMax/1 -> Divide1/2, Product3/2, Divide/1
  MinMax1/1 -> Divide/2
  Constant/1 -> Product2/1
  Constant1/1 -> Product2/2
  Product2/1 -> Divide1/1
  Divide/1 -> Mux/2  "C_R"
  Divide1/1 -> Mux/1  "NTU"
  Mux/1 -> Effectivness/1
  t_1_A/1 -> Mux2/1, Sum/1
  m_1_W/1 -> Product/2, Mux1/2, m_2_W/1
  Sum/1 -> Product3/1
  Effectivness/1 -> Product4/2
  Product3/1 -> Product4/1
  Product4/1 -> Mux2/4, Mux1/4
  t_2_w/1 -> t_2_W/1
  Mux1/1 -> t_2_w/1
  Mux2/1 -> t_2_a/1
  t_2_a/1 -> t_2_A/1

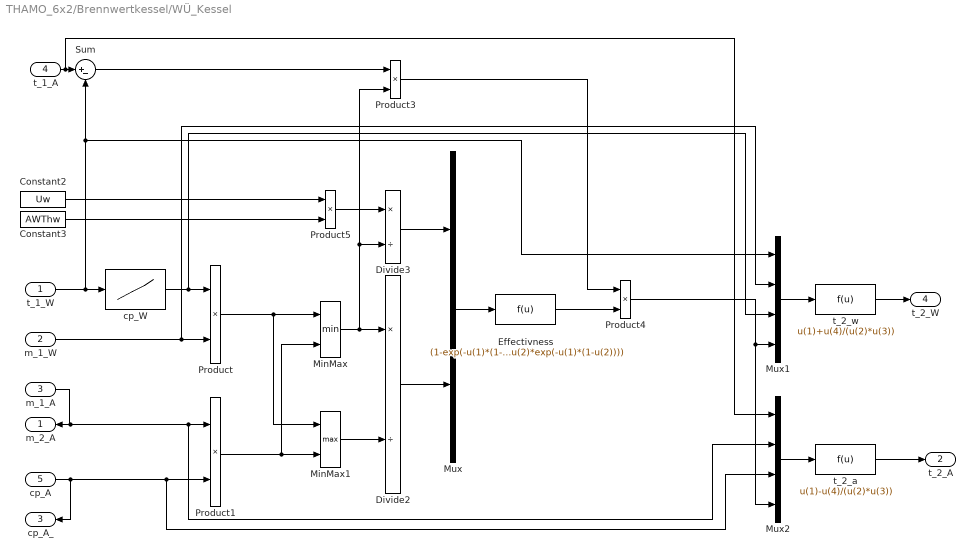
== system THAMO_6x2/Brennwertkessel/WÜ_Kessel ==
  t_1_W : Inport
  m_1_W : Inport  Port=2
  m_1_A : Inport  Port=3
  t_1_A : Inport  Port=4
  cp_A : Inport  Port=5
  Constant2 : Constant  Value=Uw
  Constant3 : Constant  Value=AWThw
  Divide2 : Product  Inputs=*/
  Divide3 : Product  Inputs=*/
  Effectivness : Fcn  Expr=(1-exp(-u(1)*(1-u(2))))/(1-u(2)*exp(-u(1)*(1-u(2))))
  MinMax : MinMax  Inputs=2
  MinMax1 : MinMax  Function=max  Inputs=2
  Mux : Mux  Inputs=2
  Mux1 : Mux
  Mux2 : Mux
  Product{,1,3..5} (5 alike) : Product
  Sum : Sum  Inputs=|+-
  cp_W : Lookup_n-D  NumberOfTableDimensions=1  BreakpointsForDimension1=[0,10,20,30,40,50,60,70,80,90,100]  Table=[4218,4192,4182,4179,4179,4181,4184,4190,4196,4205,4216]  InternalRulePriority=Speed  RndMeth=Simplest  InputSameDT=on
  t_2_a : Fcn  Expr=u(1)-u(4)/(u(2)*u(3))
  t_2_w : Fcn  Expr=u(1)+u(4)/(u(2)*u(3))
  m_2_A : Outport
  t_2_A : Outport  Port=2
  cp_A_ : Outport  Port=3
  t_2_W : Outport  Port=4
  wires:
  cp_A/1 -> Mux2/3, Product1/2, cp_A_/1
  m_1_A/1 -> Mux2/2, Product1/1, m_2_A/1
  Mux1/1 -> t_2_w/1
  Sum/1 -> Product3/1
  Product1/1 -> MinMax/2, MinMax1/2
  Product/1 -> MinMax1/1, MinMax/1
  cp_W/1 -> Mux1/3, Product/1
  t_1_W/1 -> Mux1/1, Sum/2, cp_W/1
  m_1_W/1 -> Mux1/2, Product/2
  MinMax/1 -> Divide3/2, Product3/2, Divide2/1
  MinMax1/1 -> Divide2/2
  Constant2/1 -> Product5/1
  Product5/1 -> Divide3/1
  Constant3/1 -> Product5/2
  Mux/1 -> Effectivness/1
  Divide3/1 -> Mux/1
  Divide2/1 -> Mux/2
  t_1_A/1 -> Mux2/1, Sum/1
  Effectivness/1 -> Product4/2
  Product3/1 -> Product4/1
  t_2_w/1 -> t_2_W/1
  Mux2/1 -> t_2_a/1
  t_2_a/1 -> t_2_A/1
  Product4/1 -> Mux1/4, Mux2/4

== system THAMO_6x2/Haupt-Pumpe/Wirkungsgrad ==
  Massenstrom : Inport
  St : Inport  Port=2
  MATLAB Function : MATLAB Function  TreatAsAtomicUnit=on
  const1 : Constant  Value=a0
  const11 : Constant  Value=a
  const2 : Constant  Value=a1
  const3 : Constant  Value=a2
  const9 : Constant  Value=eta_max
  eta : Outport
  wires:
  St/1 -> MATLAB Function/7(St)
  const2/1 -> MATLAB Function/2(a1)
  const1/1 -> MATLAB Function/1(a0)
  const3/1 -> MATLAB Function/3(a2)
  const9/1 -> MATLAB Function/4(eta_N)
  const11/1 -> MATLAB Function/5(a)
  Massenstrom/1 -> MATLAB Function/6(m)
  MATLAB Function/1(eta) -> eta/1

== system THAMO_6x2/Haupt-Pumpe/basic_THB ==
  Bus Creator : BusCreator  InitFcn=load THB.mat  Inputs=14  OutDataTypeStr=Bus: THB
  const1 : Constant  Value=hgt
  const2 : Constant  Value=mix2
  const21 : Constant  Value=ID  mask{mID=Pressure Drop from Massflow}
      mask prompts: mID "ID for pressure drop calculation"
      mask init:
      | ID = (mID-1)*10000+1;
      mask TypeOptions mID: No Pressure Drop | Pressure Drop from Massflow | Full Pressure Drop with Static Height
  const{22..23,30..31} (4 alike) : Constant  Value=0
  const24 : Constant  Value=t
  const25 : Constant  Value=mdot
  const26 : Constant  Value=p
  const27 : Constant  Value=fluid  mask{fluid=Water}
      mask TypeOptions fluid: Water | Air | Cotton Oil | Silicone Oil | Water-Glycol Mix | Tyfocor LS | Water (Constant 20°C) | Air (dry+ constant 20°C)
  const28 : Constant  Value=mix
  const29 : Constant  Value=dia
  const3 : Constant  Value=mix3
  THB : Outport
  wires:
  const3/1 -> Bus Creator/8  "FluidMix3"
  const2/1 -> Bus Creator/7  "FluidMix2"
  const1/1 -> Bus Creator/14  "GeodeticHeight"
  const31/1 -> Bus Creator/13  "HydraulicInductance"
  const23/1 -> Bus Creator/12  "DPQuadratic"
  const22/1 -> Bus Creator/11  "DPLinear"
  const29/1 -> Bus Creator/9  "DiameterLastPiece"
  const30/1 -> Bus Creator/10  "DPConstant"
  Bus Creator/1 -> THB/1
  const21/1 -> Bus Creator/1  "ID"
  const24/1 -> Bus Creator/2  "Temperature"
  const25/1 -> Bus Creator/3  "MassFlow"
  const26/1 -> Bus Creator/4  "Pressure"
  const27/1 -> Bus Creator/5  "FluidType"
  const28/1 -> Bus Creator/6  "FluidMix"

== system THAMO_6x2/Haupt-Pumpe/thermal_capacity ==
  Tin : Inport
  mdot : Inport  Port=2
  1/(m*cp) : Gain  Gain=1/mcp  SaturateOnIntegerOverflow=on  OutDataTypeStr=Inherit: Same as input  ParamDataTypeStr=Inherit: Same as input
  Integrator : Integrator  InitialCondition=20
  Product1 : Product  Inputs=3  SaturateOnIntegerOverflow=on  InputSameDT=on  OutDataTypeStr=Inherit: Same as first input
  Sum1 : Sum  Inputs=-+  SaturateOnIntegerOverflow=on  InputSameDT=on  OutDataTypeStr=Inherit: Same as first input
  cp1 : Lookup_n-D  NumberOfTableDimensions=1  BreakpointsForDimension1=[0,10,20,30,40,50,60,70,80,90,100]  Table=[4218,4192,4182,4179,4179,4181,4184,4190,4196,4205,4216]  InternalRulePriority=Speed  RndMeth=Simplest  InputSameDT=on
  Tout : Outport
  wires:
  mdot/1 -> Product1/2
  Tin/1 -> cp1/1, Sum1/2
  Integrator/1 -> Sum1/1, Tout/1
  Product1/1 -> 1/(m*cp)/1
  1/(m*cp)/1 -> Integrator/1
  Sum1/1 -> Product1/1
  cp1/1 -> Product1/3

== system THAMO_6x2/Hydr. Weiche/MEAN ==
  T_VL : Inport
  T_RL : Inport  Port=2
  Fcn : Fcn  Expr=(u(1)+u(2))/2
  Mux : Mux  Inputs=2
  Tm : Outport
  wires:
  T_RL/1 -> Mux/2
  Fcn/1 -> Tm/1
  Mux/1 -> Fcn/1
  T_VL/1 -> Mux/1

== system THAMO_6x2/Mischer/Ventil ==
  note: Berechnung kv aus St
      | Umrechnung kv in qua
  note: Ventillaufzeit
  THB__1_W : Inport
  St : Inport  Port=2
  Bus Assignment : BusAssignment  AssignedSignals=Pressure,DPConstant,DPLinear,DPQuadratic
  Bus Selector : BusSelector  OutputSignals=MassFlow,Pressure
  Bus Selector1 : BusSelector  OutputSignals=DPConstant,DPLinear,DPQuadratic  OutputAsBus=on
  Demux : Demux  Outputs=3
  Rate Limiter : RateLimiter  RisingSlewLimit=1/dt_V  FallingSlewLimit=-1/dt_V  SampleTimeMode=inherited
  Ventilkennlinie : Subsystem
  pressuredrop : Subsystem  mask(pressure drop){}
      mask help:
      | Pressure drop according to input values of con, lin and qua:
      | dp = con + lin*mdot + qua*mdot²
      | The coefficients are also added to the correponding THB elements.
      mask Help: web(fullfile(path_carnot('help'),'Pressuredrop.html'),'-helpbrowser')
  THB__2_W : Outport
  wires:
  Rate Limiter/1 -> Ventilkennlinie/1(St)
  Ventilkennlinie/1(qua) -> pressuredrop/4(qua)
  Demux/1 -> Bus Assignment/3
  Bus Assignment/1 -> THB__2_W/1
  THB__1_W/1 -> Bus Assignment/1, Ventilkennlinie/2(THB__1_W), Bus Selector1/1, Bus Selector/1
  St/1 -> Rate Limiter/1
  pressuredrop/2(clq_out) -> Demux/1  "clq"
  Bus Selector/2 -> pressuredrop/2(p_in)  "<Pressure>"
  Bus Selector/1 -> pressuredrop/1(mdot)  "<MassFlow>"
  pressuredrop/1(p_out) -> Bus Assignment/2  "p"
  Bus Selector1/1 -> pressuredrop/3(clq_in)  "clq"
  Demux/2 -> Bus Assignment/4
  Demux/3 -> Bus Assignment/5

== system THAMO_6x2/Mischer/Ventil1 ==
  note: Berechnung kv aus St
      | Umrechnung kv in qua
  note: Ventillaufzeit
  THB__1_W : Inport
  St : Inport  Port=2
  Bus Assignment : BusAssignment  AssignedSignals=Pressure,DPConstant,DPLinear,DPQuadratic
  Bus Selector : BusSelector  OutputSignals=MassFlow,Pressure
  Bus Selector1 : BusSelector  OutputSignals=DPConstant,DPLinear,DPQuadratic  OutputAsBus=on
  Demux : Demux  Outputs=3
  Rate Limiter : RateLimiter  RisingSlewLimit=1/dt_V  FallingSlewLimit=-1/dt_V  SampleTimeMode=inherited
  Ventilkennlinie : Subsystem
  pressuredrop : Subsystem  mask(pressure drop){}
      mask help:
      | Pressure drop according to input values of con, lin and qua:
      | dp = con + lin*mdot + qua*mdot²
      | The coefficients are also added to the correponding THB elements.
      mask Help: web(fullfile(path_carnot('help'),'Pressuredrop.html'),'-helpbrowser')
  THB__2_W : Outport
  wires:
  Rate Limiter/1 -> Ventilkennlinie/1(St)
  Ventilkennlinie/1(qua) -> pressuredrop/4(qua)
  Demux/1 -> Bus Assignment/3
  Bus Assignment/1 -> THB__2_W/1
  THB__1_W/1 -> Bus Assignment/1, Ventilkennlinie/2(THB__1_W), Bus Selector1/1, Bus Selector/1
  St/1 -> Rate Limiter/1
  pressuredrop/2(clq_out) -> Demux/1  "clq"
  Bus Selector/2 -> pressuredrop/2(p_in)  "<Pressure>"
  Bus Selector/1 -> pressuredrop/1(mdot)  "<MassFlow>"
  pressuredrop/1(p_out) -> Bus Assignment/2  "p"
  Bus Selector1/1 -> pressuredrop/3(clq_in)  "clq"
  Demux/2 -> Bus Assignment/4
  Demux/3 -> Bus Assignment/5

== system THAMO_6x2/Rohr/Druckverlust ==
  THB__1_W : Inport
  Bus Selector : BusSelector  OutputSignals=MassFlow,Pressure
  Bus Selector1 : BusSelector  OutputSignals=DPConstant,DPLinear,DPQuadratic  OutputAsBus=on
  Bus Selector2 : BusSelector  OutputSignals=GeodeticHeight  OutputAsBus=on
  Bus Selector3 : BusSelector  OutputSignals=Temperature
  Constant : Constant  Value=H
  Constant1 : Constant  Value=9.81
  Constant2 : Constant  Value=0
  Demux : Demux  Outputs=3
  Pressuredrop : Subsystem  mask(pressure drop){}
      mask help:
      | Pressure drop according to input values of con, lin and qua:
      | dp = con + lin*mdot + qua*mdot²
      | The coefficients are also added to the correponding THB elements.
      mask Help: web(fullfile(path_carnot('help'),'Pressuredrop.html'),'-helpbrowser')
  Product : Product  Inputs=3
  Sum : Sum  Inputs=++|
  dp einfach : Subsystem
  rho : Lookup_n-D  NumberOfTableDimensions=1  BreakpointsForDimension1=[0,10,20,30,40,50,60,70,80,90,100]  Table=[999.84,999.7,998.2,995.64,992.21,988.03,983.19,977.76,971.79,965.3,958.35]  InternalRulePriority=Speed  RndMeth=Simplest  InputSameDT=on
  p_2_W : Outport
  dpc_2_W : Outport  Port=2
  dpl_2_W : Outport  Port=3
  dpq_2_W : Outport  Port=4
  Hgeo_2_W : Outport  Port=5
  wires:
  Bus Selector/2 -> Pressuredrop/2(p_in)  "<Pressure>"
  Bus Selector/1 -> Pressuredrop/1(mdot)  "<MassFlow>"
  Bus Selector1/1 -> Pressuredrop/3(clq_in)
  THB__1_W/1 -> Bus Selector3/1, Bus Selector2/1, dp einfach/1(THB__1_W), Bus Selector1/1, Bus Selector/1
  Pressuredrop/1(p_out) -> p_2_W/1
  Demux/1 -> dpc_2_W/1
  Demux/2 -> dpl_2_W/1
  Demux/3 -> dpq_2_W/1
  Pressuredrop/2(clq_out) -> Demux/1
  Constant/1 -> Sum/1, Product/3
  Sum/1 -> Hgeo_2_W/1
  Product/1 -> Pressuredrop/4(con)
  rho/1 -> Product/2
  Constant1/1 -> Product/1
  Bus Selector2/1 -> Sum/2
  Constant2/1 -> Pressuredrop/5(lin)
  dp einfach/1(qua) -> Pressuredrop/6(qua)
  Bus Selector3/1 -> rho/1  "<Temperature>"

== system THAMO_6x2/Rohr/Wärmeverlust ==
  THB__1_W : Inport
  t___L : Inport  Port=2
  Add : Sum  Inputs=-+
  Add1 : Sum  Inputs=-+
  Add2 : Sum  Inputs=+-
  Bus Selector : BusSelector  OutputSignals=Temperature,MassFlow
  Constant : Constant  Value=L
  Constant1 : Constant  Value=Uw
  Constant2 : Constant  Value=L
  Constant3 : Constant  Value=d
  Divide : Product  Inputs=*//
  Integrator : Integrator  InitialCondition=20
  Mux : Mux  Inputs=2
  Product : Product
  Product1 : Product  Inputs=3
  Product2 : Product
  Product3 : Product
  V : Fcn  Expr=((u(2)/1000)^2*3.1415/4)*u(1)
  cp_W : Lookup_n-D  NumberOfTableDimensions=1  BreakpointsForDimension1=[0,10,20,30,40,50,60,70,80,90,100]  Table=[4218,4192,4182,4179,4179,4181,4184,4190,4196,4205,4216]  InternalRulePriority=Speed  RndMeth=Simplest  InputSameDT=on
  rho : Lookup_n-D  NumberOfTableDimensions=1  BreakpointsForDimension1=[0,10,20,30,40,50,60,70,80,90,100]  Table=[999.84,999.7,998.2,995.64,992.21,988.03,983.19,977.76,971.79,965.3,958.35]  InternalRulePriority=Speed  RndMeth=Simplest  InputSameDT=on
  t_2_W : Outport
  wires:
  THB__1_W/1 -> Bus Selector/1
  Bus Selector/1 -> cp_W/1, rho/1, Add/2  "<Temperature>"
  Bus Selector/2 -> Product1/2  "<MassFlow>"
  Constant1/1 -> Product/2
  Constant/1 -> Product/1
  cp_W/1 -> Divide/2, Product1/3
  Add/1 -> Product1/1
  Product1/1 -> Add1/2
  Constant2/1 -> Mux/1
  Constant3/1 -> Mux/2
  Mux/1 -> V/1
  rho/1 -> Product2/1
  V/1 -> Product2/2
  Product2/1 -> Divide/3
  Add1/1 -> Divide/1
  Divide/1 -> Integrator/1
  Integrator/1 -> Add2/1, Add/1, t_2_W/1
  t___L/1 -> Add2/2
  Add2/1 -> Product3/2
  Product3/1 -> Add1/1
  Product/1 -> Product3/1

== system THAMO_6x2/Stufenloser Regler/PID-controller-he ==
  e : Inport
  Derivative : Derivative
  Integrator : Integrator  LimitOutput=on  UpperSaturationLimit=1  LowerSaturationLimit=0
  Kd : Gain  Gain=Kd
  Ki : Gain  Gain=Ki
  Kp : Gain  Gain=Kp
  Saturation : Saturate  UpperLimit=1  LowerLimit=0
  Sum1 : Sum  Inputs=+++
  u : Outport
  wires:
  Derivative/1 -> Sum1/3
  Ki/1 -> Integrator/1
  Kp/1 -> Sum1/1
  Kd/1 -> Derivative/1
  Saturation/1 -> u/1
  Sum1/1 -> Saturation/1
  e/1 -> Kd/1, Ki/1, Kp/1
  Integrator/1 -> Sum1/2

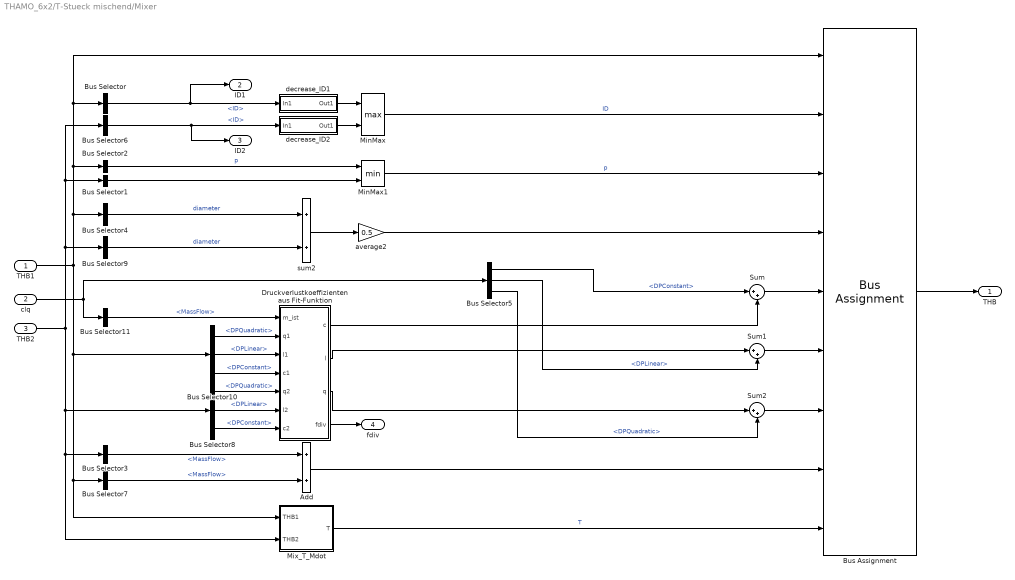
== system THAMO_6x2/T-Stueck mischend/Mixer ==
  THB1 : Inport
  clq : Inport  Port=2
  THB2 : Inport  Port=3
  Add : Sum
  Bus Assignment : BusAssignment  AssignedSignals=ID,Pressure,DiameterLastPiece,DPConstant,DPLinear,DPQuadratic,MassFlow,Temperature
  Bus Selector : BusSelector  OutputSignals=ID
  Bus Selector1 : BusSelector  OutputSignals=Pressure  OutputAsBus=on
  Bus Selector10 : BusSelector  OutputSignals=DPQuadratic,DPLinear,DPConstant
  Bus Selector2 : BusSelector  OutputSignals=Pressure  OutputAsBus=on
  Bus Selector4 : BusSelector  OutputSignals=DiameterLastPiece  OutputAsBus=on
  Bus Selector5 : BusSelector  OutputSignals=DPConstant,DPLinear,DPQuadratic
  Bus Selector6 : BusSelector  OutputSignals=ID
  Bus Selector8 : BusSelector  OutputSignals=DPQuadratic,DPLinear,DPConstant
  Bus Selector9 : BusSelector  OutputSignals=DiameterLastPiece  OutputAsBus=on
  Bus Selector11 : BusSelector  OutputSignals=MassFlow
  Bus Selector3 : BusSelector  OutputSignals=MassFlow
  Bus Selector7 : BusSelector  OutputSignals=MassFlow
  Druckverlustkoeffizienten aus Fit-Funktion : MATLAB Function  TreatAsAtomicUnit=on
  MinMax : MinMax  Function=max  Inputs=2
  MinMax1 : MinMax  Inputs=2
  Mix_T_Mdot : Subsystem  mask(mix_temperature){mixcalc=Tmix = (mdot1*T1 + mdot2*T2)/(mdot1+mdot2)}
      mask prompts: mixcalc "Calculation of mixture :"
      mask help:
      | Calculate the temperature of the mixture of two flows. Uses enthalpy balance for humid air. Liquids may be mixed by the (faster and approximate) equation:
      | Tmix = (mdot1*T1 + mdot2*T2)/(mdot1+mdot2)
      mask Help: web(fullfile(path_carnot('help'),'Mix_T_Mdot.html'),'-helpbrowser')
      mask TypeOptions mixcalc: Tmix = (mdot1*T1 + mdot2*T2)/(mdot1+mdot2) | Enthalpy balance
  Sum : Sum  Inputs=|++
  Sum1 : Sum  Inputs=|++
  Sum2 : Sum  Inputs=|++
  average2 : Gain  Gain=0.5  SaturateOnIntegerOverflow=on  OutDataTypeStr=Inherit: Same as input  ParamDataTypeStr=Inherit: Same as input
  decrease_ID1 : Subsystem
  decrease_ID2 : Subsystem
  sum2 : Sum  SaturateOnIntegerOverflow=on  InputSameDT=on  OutDataTypeStr=Inherit: Same as first input
  THB : Outport
  ID1 : Outport  Port=2
  ID2 : Outport  Port=3
  fdiv : Outport  Port=4
  wires:
  Bus Selector10/1 -> Druckverlustkoeffizienten aus Fit-Funktion/2(q1)  "<DPQuadratic>"
  THB2/1 -> Bus Selector6/1, Bus Selector1/1, Bus Selector9/1, Bus Selector8/1, Bus Selector3/1, Mix_T_Mdot/2(THB2)
  THB1/1 -> Bus Selector10/1, Bus Selector7/1, Mix_T_Mdot/1(THB1), Bus Assignment/1, Bus Selector/1, Bus Selector2/1, Bus Selector4/1
  Bus Selector6/1 -> ID2/1, decrease_ID2/1(In1)  "<ID>"
  Add/1 -> Bus Assignment/8
  MinMax/1 -> Bus Assignment/2  "ID"
  sum2/1 -> average2/1
  Bus Selector8/3 -> Druckverlustkoeffizienten aus Fit-Funktion/7(c2)  "<DPConstant>"
  Bus Selector2/1 -> MinMax1/1  "p"
  Bus Selector7/1 -> Add/2  "<MassFlow>"
  decrease_ID1/1(Out1) -> MinMax/1
  Mix_T_Mdot/1(T) -> Bus Assignment/9  "T"
  Bus Selector3/1 -> Add/1  "<MassFlow>"
  MinMax1/1 -> Bus Assignment/3  "p"
  Druckverlustkoeffizienten aus Fit-Funktion/4(fdiv) -> fdiv/1
  Bus Selector10/3 -> Druckverlustkoeffizienten aus Fit-Funktion/4(c1)  "<DPConstant>"
  Bus Selector10/2 -> Druckverlustkoeffizienten aus Fit-Funktion/3(l1)  "<DPLinear>"
  clq/1 -> Bus Selector5/1, Bus Selector11/1
  Bus Selector8/1 -> Druckverlustkoeffizienten aus Fit-Funktion/5(q2)  "<DPQuadratic>"
  Bus Selector11/1 -> Druckverlustkoeffizienten aus Fit-Funktion/1(m_ist)  "<MassFlow>"
  Bus Selector4/1 -> sum2/1  "diameter"
  Bus Selector1/1 -> MinMax1/2
  Bus Selector9/1 -> sum2/2  "diameter"
  Bus Selector8/2 -> Druckverlustkoeffizienten aus Fit-Funktion/6(l2)  "<DPLinear>"
  average2/1 -> Bus Assignment/4
  decrease_ID2/1(Out1) -> MinMax/2
  Bus Selector/1 -> ID1/1, decrease_ID1/1(In1)  "<ID>"
  Bus Assignment/1 -> THB/1
  Bus Selector5/1 -> Sum/1  "<DPConstant>"
  Druckverlustkoeffizienten aus Fit-Funktion/1(c) -> Sum/2
  Sum/1 -> Bus Assignment/5
  Sum1/1 -> Bus Assignment/6
  Sum2/1 -> Bus Assignment/7
  Druckverlustkoeffizienten aus Fit-Funktion/2(l) -> Sum1/1
  Druckverlustkoeffizienten aus Fit-Funktion/3(q) -> Sum2/1
  Bus Selector5/2 -> Sum1/2  "<DPLinear>"
  Bus Selector5/3 -> Sum2/2  "<DPQuadratic>"

== system THAMO_6x2/T-Stueck mischend/PT1_for_fdiv ==
  ID_1 : Inport
  ID_2 : Inport  Port=2
  fdiv : Inport  Port=3
  Compare To Zero : simulink/Logic and Bit Operations/Compare To Zero  relop=<=  OutDataTypeStr=uint8
  Compare To Zero1 : simulink/Logic and Bit Operations/Compare To Zero  relop=<=  OutDataTypeStr=uint8
  Constant : Constant  Value=0
  Constant1 : Constant
  Gain1 : Gain  Gain=2
  Index Vector : MultiPortSwitch  DataPortOrder=Zero-based contiguous  zeroidx=on
  Memory : Memory
  MinMax2 : MinMax  Function=max  Inputs=2
  f_div : Outport
  wires:
  fdiv/1 -> Memory/1
  Compare To Zero1/1 -> Gain1/1
  Compare To Zero/1 -> MinMax2/1
  MinMax2/1 -> Index Vector/1
  ID_1/1 -> Compare To Zero/1
  ID_2/1 -> Compare To Zero1/1
  Constant/1 -> Index Vector/3
  Memory/1 -> Index Vector/2
  Constant1/1 -> Index Vector/4
  Gain1/1 -> MinMax2/2
  Index Vector/1 -> f_div/1

== system THAMO_6x2/T-Stueck trennend/increase_ID ==
  In1 : Inport
  Abs : Abs
  Bias : Bias  Bias=1
  Dot Product1 : DotProduct  InputSameDT=on  OutDataTypeStr=Inherit: Inherit via internal rule
  Sign : Signum
  Out1 : Outport
  wires:
  Bias/1 -> Dot Product1/2
  Sign/1 -> Dot Product1/1
  Abs/1 -> Bias/1
  Dot Product1/1 -> Out1/1
  In1/1 -> Sign/1, Abs/1

== system THAMO_6x2/Ventil/Ventilkennlinie ==
  St : Inport
  THB__1_W : Inport  Port=2
  Bus Selector : BusSelector  OutputSignals=Temperature
  Constant2 : Constant  Value=ART
  Constant6 : Constant  Value=n_0
  Constant8 : Constant  Value=kvs
  GLP : Fcn  Expr=u(2)*((1/u(2))^u(1))
  Mux : Mux  Inputs=2
  Mux2 : Mux  Inputs=2
  Mux3 : Mux  Inputs=2
  Product : Product
  Switch : Switch  Criteria=u2 > Threshold  Threshold=1
  calc_qua_kvs : Fcn  Expr=(3600^2*100)/(u(1)^2*u(2))
  linear : Fcn  Expr=u(2)+(1-u(2))*u(1)
  rho : Lookup_n-D  NumberOfTableDimensions=1  BreakpointsForDimension1=[0,10,20,30,40,50,60,70,80,90,100]  Table=[999.84,999.7,998.2,995.64,992.21,988.03,983.19,977.76,971.79,965.3,958.35]  InternalRulePriority=Speed  RndMeth=Simplest  InputSameDT=on
  qua : Outport
  wires:
  Bus Selector/1 -> rho/1  "<Temperature>"
  St/1 -> Mux2/1, Mux3/1
  linear/1 -> Switch/3
  Mux2/1 -> GLP/1
  Mux3/1 -> linear/1
  Constant6/1 -> Mux2/2, Mux3/2
  Constant8/1 -> Product/2
  Switch/1 -> Product/1
  Constant2/1 -> Switch/2
  GLP/1 -> Switch/1
  THB__1_W/1 -> Bus Selector/1
  calc_qua_kvs/1 -> qua/1
  Mux/1 -> calc_qua_kvs/1
  Product/1 -> Mux/1
  rho/1 -> Mux/2
